simulink model "control_system_observer"  (R2022a)
settings: Solver=FixedStepDiscrete  StartTime=0.0  StopTime=t3(end)  RelTol=1e-3
values from neighbouring files (symbols this model uses):
  A = [-1/tau1 -AOL/tau1 ... (first row only)    [observer_test.m]    (also in series_res_comp_test.m = [-1/(Rsa*Cma) 0; 0 -1/(Rcc*Ccc)]*Ts*1e-6 + [1 0; 0 1])
  B = [0; (R3*g)/(tau2*R4*(AOL*(1-rho)+g))]    [observer_test.m]    (also in series_res_comp_test.m = [1/(Rsa*Cma); 1/(Rcc*Ccc)]*Ts*1e-6)
  Cmeas = [-1/Rsa -1/Rcc]    [series_res_comp_test.m]
  Dmeas = (1/Rsa + 1/Rcc)    (= 0.0011404494382)    [series_res_comp_test.m]
  L = place(A',C',pObs)'    [observer_test.m]    (also in series_res_comp_test.m = place(A',Cmeas',pObs)'*Ts*1e-6)
  Ts = 1e-6    (= 1e-06)    [observer_test.m]    (also in series_res_comp_test.m = 1)
undefined symbols (not defined in the file or in its folder): DiscIntNeverNeededParam
settings Model: Creator=iande  LastModifiedBy=iande

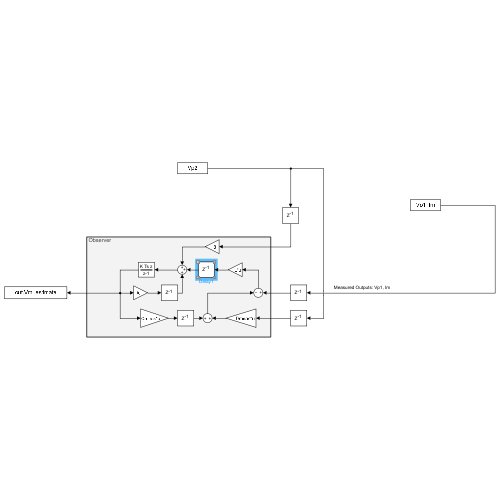
[thumbnail: Simulink's stored preview of the top-level diagram]
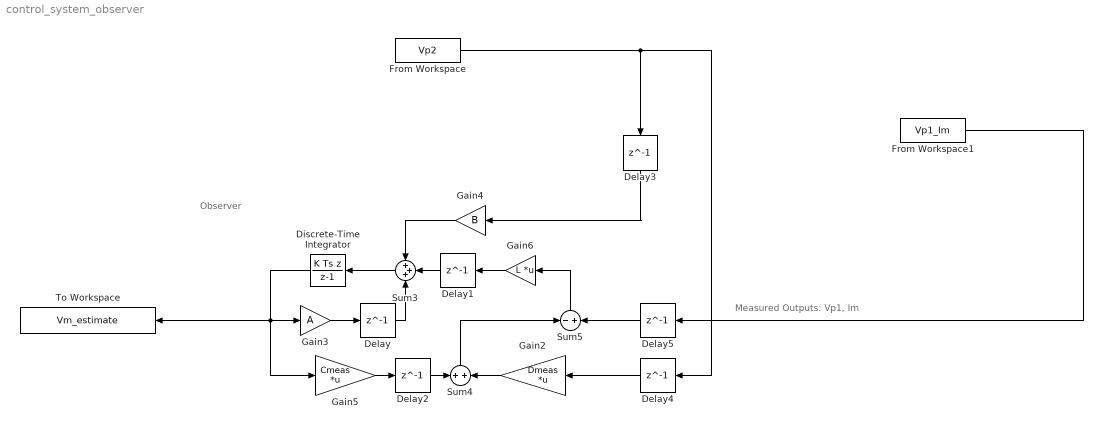
== system control_system_observer ==
  note: Measured Outputs: Vp1, Im
  note: Observer
  Delay{,1..5} (6 alike) : Delay  DelayLength=1  InitialCondition=0  SampleTime=Ts
  Discrete-Time Integrator : DiscreteIntegrator  IntegratorMethod=Integration: Backward Euler  SampleTime=Ts  ICPrevOutput=DiscIntNeverNeededParam  ICPrevScaledInput=DiscIntNeverNeededParam
  From Workspace : FromWorkspace  VariableName=Vp2  SampleTime=Ts
  From Workspace1 : FromWorkspace  VariableName=Vp1_Im  SampleTime=Ts
  Gain2 : Gain  Gain=Dmeas  Multiplication=Matrix(K*u)
  Gain3 : Gain  Gain=A
  Gain4 : Gain  Gain=B
  Gain5 : Gain  Gain=Cmeas  Multiplication=Matrix(K*u)
  Gain6 : Gain  Gain=L  Multiplication=Matrix(K*u)
  Sum3 : Sum  Inputs=+++
  Sum4 : Sum
  Sum5 : Sum  Inputs=-+
  To Workspace : ToWorkspace  VariableName=Vm_estimate  SaveFormat=Timeseries  SampleTime=-1
  wires:
  Gain3/1 -> Delay/1
  Discrete-Time Integrator/1 -> To Workspace/1, Gain5/1, Gain3/1
  Sum5/1 -> Gain6/1
  From Workspace/1 -> Delay4/1, Delay3/1
  Gain5/1 -> Delay2/1
  Gain2/1 -> Sum4/2
  Sum4/1 -> Sum5/1
  Gain6/1 -> Delay1/1
  From Workspace1/1 -> Delay5/1
  Gain4/1 -> Sum3/1
  Sum3/1 -> Discrete-Time Integrator/1
  Delay/1 -> Sum3/3
  Delay1/1 -> Sum3/2
  Delay2/1 -> Sum4/1
  Delay3/1 -> Gain4/1
  Delay4/1 -> Gain2/1
  Delay5/1 -> Sum5/2
